simulink model "CapstoneUpdated"  (R2021b)
settings: Solver=VariableStepAuto  StartTime=0.0  StopTime=10.0  RelTol=1e-3
settings Model: Creator=davidedelson  LastModifiedBy=davidedelson
settings SolverCC: AlgebraicLoopSolver=TrustRegion
settings DebuggingCC: SFMachineParentedDataDiag=warning

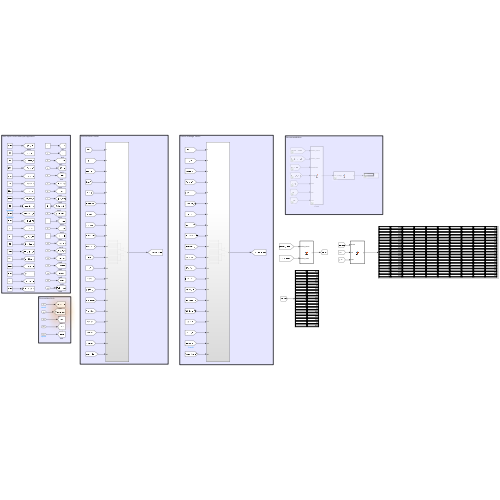
[thumbnail: Simulink's stored preview of the top-level diagram]
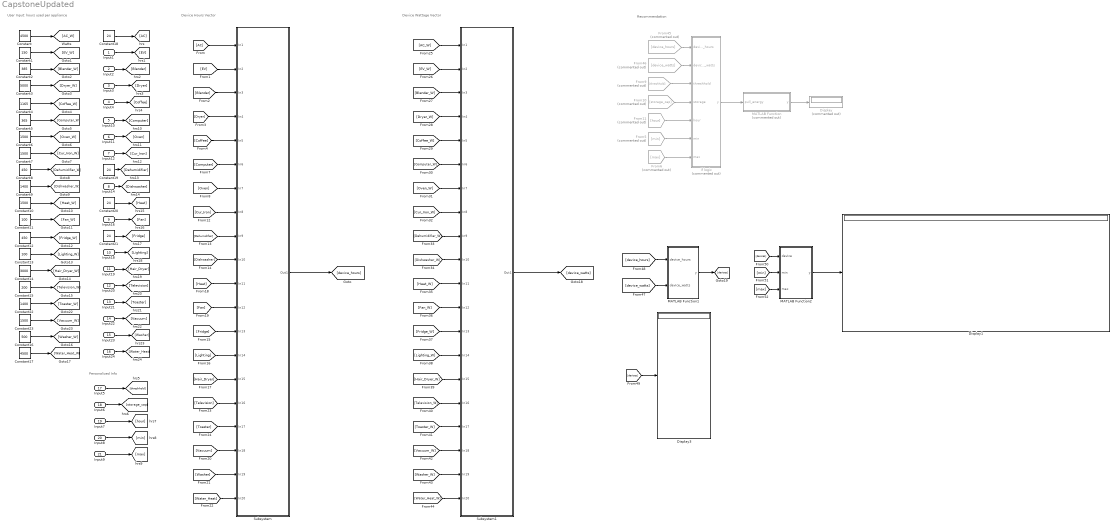
== system CapstoneUpdated ==
  note: Device Wattage Vector
  note: Device Hours Vector
  note: Recommendation
  note: User Input: hours used per appliance
  note: Personalized Info
  Input1 : Inport
  Input2 : Inport  Port=2
  Input3 : Inport  Port=3
  Input4 : Inport  Port=4
  Input10 : Inport  Port=5
  Input11 : Inport  Port=6
  Input12 : Inport  Port=7
  Input14 : Inport  Port=8
  Input16 : Inport  Port=9
  Input18 : Inport  Port=10
  Input19 : Inport  Port=11
  Input20 : Inport  Port=12
  Input21 : Inport  Port=13
  Input22 : Inport  Port=14
  Input23 : Inport  Port=15
  Input24 : Inport  Port=16
  Input5 : Inport  Port=17
  Input6 : Inport  Port=18
  Input7 : Inport  Port=19
  Input8 : Inport  Port=20
  Input9 : Inport  Port=21
  Constant : Constant  Value=4500
  Constant1 : Constant  Value=150
  Constant{6..7,10,23} (4 alike) : Constant  Value=1500
  Constant11 : Constant  Value=100
  Constant12 : Constant  Value=450
  Constant13 : Constant  Value=100
  Constant14 : Constant  Value=3000
  Constant15 : Constant  Value=200
  Constant16 : Constant  Value=500
  Constant17 : Constant  Value=4500
  Constant{18..21} (4 alike) : Constant  Value=24
  Constant2 : Constant  Value=385
  Constant22 : Constant  Value=1400
  Constant3 : Constant  Value=5000
  Constant4 : Constant  Value=1165
  Constant5 : Constant  Value=365
  Constant8 : Constant  Value=450
  Constant9 : Constant  Value=1400
  Display : Display  Commented=on
  Display1 : Display
  Display3 : Display
  From10 : From  Commented=on  GotoTag=storage_cap
  From11 : From  Commented=on  GotoTag=hour
  From45 : From  Commented=on  GotoTag=device_hours
  From46 : From  Commented=on  GotoTag=device_watts
  From5 : From  Commented=on  GotoTag=min
  From6 : From  Commented=on  GotoTag=max
  From9 : From  Commented=on  GotoTag=threshhold
  MATLAB Function : MATLAB Function  Commented=on  TreatAsAtomicUnit=on
  MATLAB Function1 : MATLAB Function  TreatAsAtomicUnit=on
  MATLAB Function2 : MATLAB Function  TreatAsAtomicUnit=on
  Subsystem : Subsystem
  Subsystem1 : Subsystem
  if logic : MATLAB Function  Commented=on  TreatAsAtomicUnit=on
  wires:
  Constant18/1 -> [AC]
  Input1/1 -> [EV]
  Input3/1 -> [Dryer]
  Input2/1 -> [Blender]
  Input4/1 -> [Coffee]
  if logic/1(y) -> MATLAB Function/1(pull_energy)
  From9/1 -> if logic/3(threshhold)
  From10/1 -> if logic/4(storage)
  From11/1 -> if logic/5(hour)
  MATLAB Function/1(y) -> Display/1
  [AC] -> Subsystem/1(In1)
  [EV] -> Subsystem/2(In2)
  [Blender] -> Subsystem/3(In3)
  [Dryer] -> Subsystem/4(In4)
  [Coffee] -> Subsystem/5(In5)
  From5/1 -> if logic/6(min)
  From6/1 -> if logic/7(max)
  Constant/1 -> [AC_W]
  Input14/1 -> [Dishwasher]
  Input10/1 -> [Computer]
  Input11/1 -> [Oven]
  Input12/1 -> [Cur_Iron]
  Input19/1 -> [Hair_Dryer]
  Constant20/1 -> [Heat]
  Input18/1 -> [Lighting]
  Input16/1 -> [Fan]
  Constant21/1 -> [Fridge]
  Input24/1 -> [Water_Heat]
  Input20/1 -> [Television]
  Input23/1 -> [Washer]
  Input21/1 -> [Toaster]
  Input22/1 -> [Vacuum]
  Constant1/1 -> [EV_W]
  Constant3/1 -> [Dryer_W]
  Constant2/1 -> [Blender_W]
  Constant5/1 -> [Computer_W]
  Constant6/1 -> [Oven_W]
  Constant7/1 -> [Cur_Iron_W]
  Constant4/1 -> [Coffee_W]
  Constant9/1 -> [Dishwasher_W]
  Constant10/1 -> [Heat_W]
  Constant13/1 -> [Lighting_W]
  Constant8/1 -> [Dehumidifier_W]
  Constant15/1 -> [Television_W]
  Constant11/1 -> [Fan_W]
  Constant14/1 -> [Hair_Dryer_W]
  Constant12/1 -> [Fridge_W]
  Constant16/1 -> [Washer_W]
  Constant22/1 -> [Toaster_W]
  Constant17/1 -> [Water_Heat_W]
  Constant23/1 -> [Vacuum_W]
  [Cur_Iron] -> Subsystem/8(In8)
  [Computer] -> Subsystem/6(In6)
  [Dehumidifier] -> Subsystem/9(In9)
  [Dishwasher] -> Subsystem/10(In10)
  [Oven] -> Subsystem/7(In7)
  [Heat] -> Subsystem/11(In11)
  [Fridge] -> Subsystem/13(In13)
  [Fan] -> Subsystem/12(In12)
  [Lighting] -> Subsystem/14(In14)
  [Hair_Dryer] -> Subsystem/15(In15)
  [Television] -> Subsystem/16(In16)
  [Vacuum] -> Subsystem/18(In18)
  [Toaster] -> Subsystem/17(In17)
  [Washer] -> Subsystem/19(In19)
  [Water_Heat] -> Subsystem/20(In20)
  Input9/1 -> [max]
  Input8/1 -> [min]
  Input7/1 -> [hour]
  Input6/1 -> [storage_cap]
  Input5/1 -> [threshhold]
  [Lighting_W] -> Subsystem1/14(In14)
  [Heat_W] -> Subsystem1/11(In11)
  [Fan_W] -> Subsystem1/12(In12)
  [Dehumidifier_W] -> Subsystem1/9(In9)
  [Television_W] -> Subsystem1/16(In16)
  [Water_Heat_W] -> Subsystem1/20(In20)
  [Washer_W] -> Subsystem1/19(In19)
  [Cur_Iron_W] -> Subsystem1/8(In8)
  [Blender_W] -> Subsystem1/3(In3)
  [AC_W] -> Subsystem1/1(In1)
  [Fridge_W] -> Subsystem1/13(In13)
  [Toaster_W] -> Subsystem1/17(In17)
  [Computer_W] -> Subsystem1/6(In6)
  [EV_W] -> Subsystem1/2(In2)
  [Vacuum_W] -> Subsystem1/18(In18)
  [Dryer_W] -> Subsystem1/4(In4)
  [Coffee_W] -> Subsystem1/5(In5)
  [Hair_Dryer_W] -> Subsystem1/15(In15)
  [Oven_W] -> Subsystem1/7(In7)
  [Dishwasher_W] -> Subsystem1/10(In10)
  Subsystem1/1(Out1) -> [device_watts]
  Subsystem/1(Out1) -> [device_hours]
  From45/1 -> if logic/1(device_hours)
  From46/1 -> if logic/2(device_watts)
  [device_watts] -> MATLAB Function1/2(device_watts)
  [device_hours] -> MATLAB Function1/1(device_hours)
  Constant19/1 -> [Dehumidifier]
  MATLAB Function1/1(y) -> [devices]
  [devices] -> Display3/1
  [devices] -> MATLAB Function2/1(device)
  [min] -> MATLAB Function2/2(min)
  [max] -> MATLAB Function2/3(max)
  MATLAB Function2/1(y) -> Display1/1

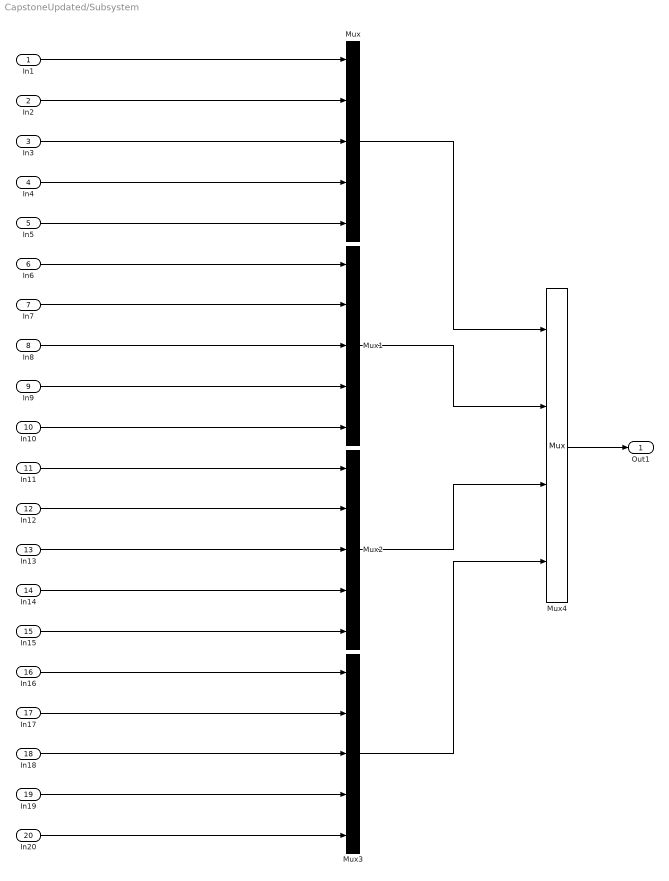
== system CapstoneUpdated/Subsystem ==
  In1 : Inport
  In2 : Inport  Port=2
  In3 : Inport  Port=3
  In4 : Inport  Port=4
  In5 : Inport  Port=5
  In6 : Inport  Port=6
  In7 : Inport  Port=7
  In8 : Inport  Port=8
  In9 : Inport  Port=9
  In10 : Inport  Port=10
  In11 : Inport  Port=11
  In12 : Inport  Port=12
  In13 : Inport  Port=13
  In14 : Inport  Port=14
  In15 : Inport  Port=15
  In16 : Inport  Port=16
  In17 : Inport  Port=17
  In18 : Inport  Port=18
  In19 : Inport  Port=19
  In20 : Inport  Port=20
  Mux{,1..3} (4 alike) : Mux  Inputs=5
  Mux4 : Mux
  Out1 : Outport
  wires:
  In1/1 -> Mux/1
  In2/1 -> Mux/2
  In3/1 -> Mux/3
  In4/1 -> Mux/4
  In5/1 -> Mux/5
  In6/1 -> Mux1/1
  In7/1 -> Mux1/2
  In8/1 -> Mux1/3
  In9/1 -> Mux1/4
  In10/1 -> Mux1/5
  In11/1 -> Mux2/1
  In12/1 -> Mux2/2
  In13/1 -> Mux2/3
  In14/1 -> Mux2/4
  In15/1 -> Mux2/5
  In16/1 -> Mux3/1
  In17/1 -> Mux3/2
  In18/1 -> Mux3/3
  In19/1 -> Mux3/4
  In20/1 -> Mux3/5
  Mux4/1 -> Out1/1
  Mux1/1 -> Mux4/2
  Mux2/1 -> Mux4/3
  Mux/1 -> Mux4/1
  Mux3/1 -> Mux4/4

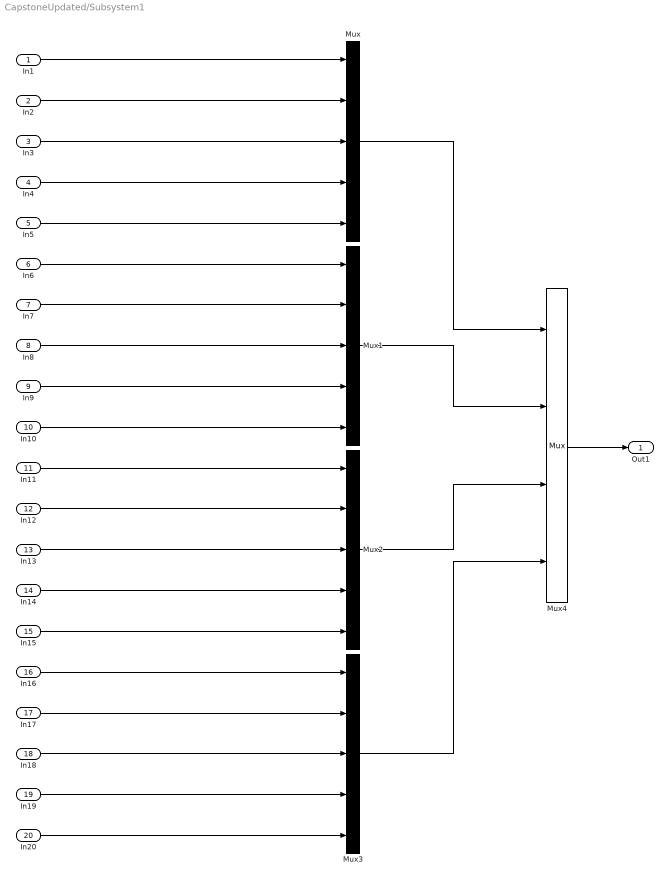
== system CapstoneUpdated/Subsystem1 ==
  In1 : Inport
  In2 : Inport  Port=2
  In3 : Inport  Port=3
  In4 : Inport  Port=4
  In5 : Inport  Port=5
  In6 : Inport  Port=6
  In7 : Inport  Port=7
  In8 : Inport  Port=8
  In9 : Inport  Port=9
  In10 : Inport  Port=10
  In11 : Inport  Port=11
  In12 : Inport  Port=12
  In13 : Inport  Port=13
  In14 : Inport  Port=14
  In15 : Inport  Port=15
  In16 : Inport  Port=16
  In17 : Inport  Port=17
  In18 : Inport  Port=18
  In19 : Inport  Port=19
  In20 : Inport  Port=20
  Mux{,1..3} (4 alike) : Mux  Inputs=5
  Mux4 : Mux
  Out1 : Outport
  wires:
  In1/1 -> Mux/1
  In2/1 -> Mux/2
  In3/1 -> Mux/3
  In4/1 -> Mux/4
  In5/1 -> Mux/5
  In6/1 -> Mux1/1
  In7/1 -> Mux1/2
  In8/1 -> Mux1/3
  In9/1 -> Mux1/4
  In10/1 -> Mux1/5
  In11/1 -> Mux2/1
  In12/1 -> Mux2/2
  In13/1 -> Mux2/3
  In14/1 -> Mux2/4
  In15/1 -> Mux2/5
  In16/1 -> Mux3/1
  In17/1 -> Mux3/2
  In18/1 -> Mux3/3
  In19/1 -> Mux3/4
  In20/1 -> Mux3/5
  Mux4/1 -> Out1/1
  Mux1/1 -> Mux4/2
  Mux2/1 -> Mux4/3
  Mux/1 -> Mux4/1
  Mux3/1 -> Mux4/4

== matlab function CapstoneUpdated/MATLAB Function ==
  data: pull_energy input; y output
function y = fcn(pull_energy)

if(pull_energy == 0)
    print("Pull Energy from Solar");
elseif(pull_energy == 1)
    print("Pull Energy from the Grid and Solar");
elseif(pull_energy == 2)
    print("Pull Energy from the Grid and Store Solar Energy");
else
    print("Pull No Energy and Store all Solar Energy");
end

y = pull_energy;

== matlab function CapstoneUpdated/if logic ==
  data: device_hours input; device_watts input; y output; threshhold input; storage input; hour input; min input; max input
function y = fcn(device_hours, device_watts, threshhold, storage, hour, min, max)

boolean has_storage;

if (storage > 0)
    has_storage = true;
else
    has_storage = false;
end

% if (has_storage == true)
%     storage_capacity = storage;
% else
%     storage_capacity = 0;
% end

watts = table2array(pvwattshourly);
m=0;
n=1;
a = zeros(24,30);
for(i=1:size(watts))
    m=m+1;
    if(m==25)
        m=1;
        n=n+1;
    end
    if(n<=30)
        a(m,n)=watts(i,2);
    end
end

b = zeros(24,1);
for(i=1:24)
    sum=0;
    for(j=1:30)
        sum = sum + a(i,j);
    end
    b(i,1) = sum/30;

    if(hour==i)
        solar_output = b(i,1);
    end
end
minPrompt = 'What is the earliest time you can do house work? ';
min = input(minPrompt);
maxPrompt = 'What is the latest time you can do house work? ';
max = input(maxPrompt);

range = fixed.Interval(min, max);
offInterval = fixed.Interval(0, 5);
midInterval1 = fixed.Interval(6, 13);
midInterval2 = fixed.Interval(19, 21);

if((overlaps(range,offInterval))||(max>=22))
    %currentCost=0.056;
    doWork
elseif((overlaps(range,midInterval1))||(overlaps(range,midInterval2)))
    %currentCost=0.087;
    doWork
else
   solar
end

t1 = hour(datetime('now','Format','HH'));
if((t1>=0 && t1<6)||(t1>=22))
    currentCost=0.056;
elseif((t1>=6 && t1<14)||(t1>=19 && t1<22))
    currentCost=0.087;
else
    currentCost=0.282;
end

if (solar_output + storage > total_output)
    decision_output = 0;
end

if (total_output > solar_output + storage)
    if (currentCost > threshhold && has_storage == false)
        decision_output = 1;
    elseif (currentCost > threshhold && has_storage == true)
        decision_output = 3;
    elseif (currentCost < threshhold && has_storage == false)
        decision_output = 1;
    else (currentCost < threshhold && has_storage == true)
        decision_output = 2;
    end
end


% Time = [hours(0:23)];
% TT = timetable(Time',[0.056;0.056;0.056;0.056;0.056;0.056;... %offpeak =12am-6am
%     0.087;0.087;0.087;0.087;0.087;0.087;0.087;0.087;... %midpeak = 6am-2pm
%     0.282;0.282;0.282;0.282;0.282;... %peak= 2-7
%     0.087;0.087;0.087;... %midpeak = 7p-10pm
%     0.056;0.056],... %offpeak =10pm -12am
%      'VariableNames',{'Prices'})

y = decision_output;

== matlab function CapstoneUpdated/MATLAB Function1 ==
  data: device_hours input; y output; device_watts input
function y = fcn(device_hours, device_watts)

device = zeros(20,2);

for i=1:20
    device(i,1) = device_hours(i);
    device(i,2) = device_watts(i);
end

y = device;

== matlab function CapstoneUpdated/MATLAB Function2 ==
  data: device input; y output; min input; max input
function y = fcn(device, min, max)

sum_usage = zeros(24,21);
counter = 1;
time = zeros(24,2);
for i=1:24
    time(i,1) = i-1;
    sum_usage(i,1) = i-1;
    for j=1:20
        if(device(j,1) == 24)
            sum_usage(i,j+1) = device(j,2);
            
            %time(i,2) = sum_usage;
        else
        
        end
    end
end

y = sum_usage;
